simulink model "closed_loop"  (R2023b)
settings: Solver=VariableStepAuto  StartTime=0.0  StopTime=0.1  RelTol=1e-3
undefined symbols (not defined in the file): a_m, config, K, K_g, K_m, K_pot
settings Model: Creator=foderking  LastModifiedBy=foderking

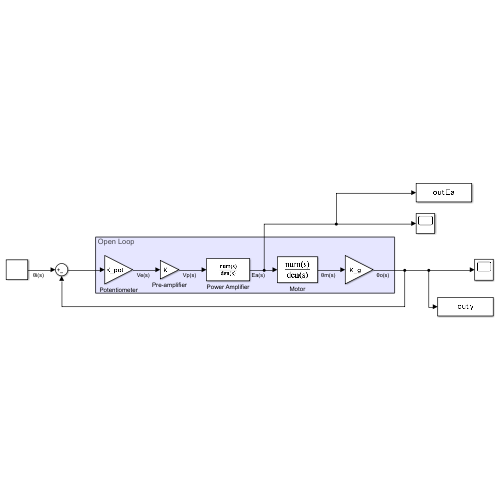
[thumbnail: Simulink's stored preview of the top-level diagram]
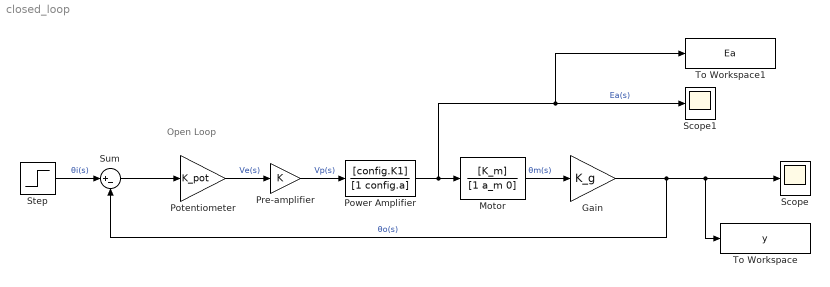
== system closed_loop ==
  note: Open Loop
  Gain : Gain  Gain=K_g
  Motor : TransferFcn  Numerator=[K_m]  Denominator=[1 a_m 0]
  Potentiometer : Gain  Gain=K_pot
  Power Amplifier : TransferFcn  Numerator=[config.K1]  Denominator=[1 config.a]
  Pre-amplifier : Gain  Gain=K
  Scope : Scope
  Scope1 : Scope
  Step : Step  Time=0  SampleTime=0
  Sum : Sum  Inputs=|+-
  To Workspace : ToWorkspace  VariableName=y  SaveFormat=Timeseries  SampleTime=-1
  To Workspace1 : ToWorkspace  VariableName=Ea  SaveFormat=Timeseries  SampleTime=-1
      settings: Save2DSignal=2-D array (concatenate along first dimension)
  wires:
  Step/1 -> Sum/1  "θi(s)"
  Gain/1 -> Sum/2, To Workspace/1, Scope/1  "θo(s)"
  Pre-amplifier/1 -> Power Amplifier/1  "Vp(s)"
  Sum/1 -> Potentiometer/1
  Motor/1 -> Gain/1  "θm(s)"
  Potentiometer/1 -> Pre-amplifier/1  "Ve(s)"
  Power Amplifier/1 -> To Workspace1/1, Scope1/1, Motor/1  "Ea(s)"
